simulink model "untitled2"  (R2024b)
settings: Solver=VariableStepAuto  StartTime=0.0  StopTime=10.0  RelTol=1e-3
undefined symbols (not defined in the file): control, Vt, zGround
libraries: uavalgslib x7
settings Model: Creator=USER  LastModifiedBy=USER

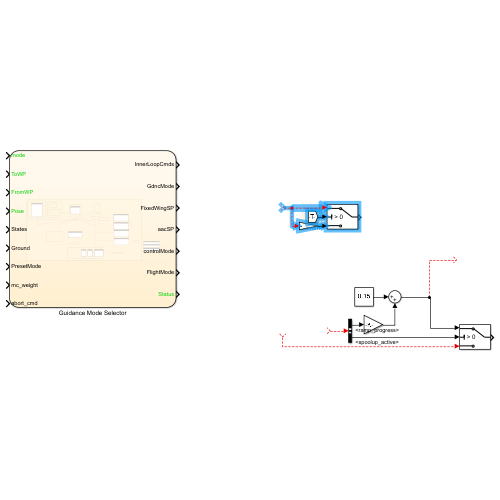
[thumbnail: Simulink's stored preview of the top-level diagram]
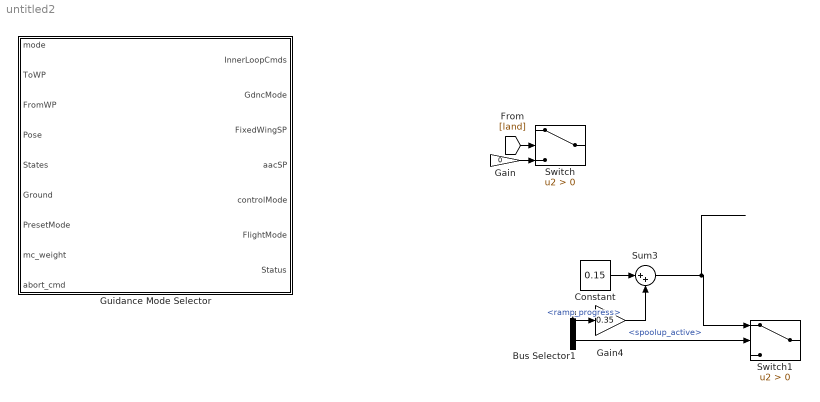
== system untitled2 ==
  Bus Selector1 : BusSelector  OutputSignals=ramp_progress,spoolup_active
  Constant : Constant  Value=0.15
  Gain : Gain  Gain=0
  Gain4 : Gain  Gain=0.35
  Guidance Mode Selector : Stateflow chart  TreatAsAtomicUnit=on
      settings: PortSchema="{\"entries\":[{\"content\":{\"sides\":[{\"content\":{\"connectorIds\":[\"In1\",\"In2\",\"In3\",\"In4\",\"In5\",\"In7\",\"In6\",\"In8\",\"In9\"]},\"type\":\"ConnectorPlacement.EquallySpacedRectSide\",\"uuid\":\"a9cfd0e2-196c-422d-b359-9161a47768c9\"},{\"content\":{\"connectorIds\":[\"Out7\",\"Out2\",\"Out4\",\"Out3\",\"Out5\",\"Out6\",\"Out1\"],\"side\":\"RIGHT\"},\"type\":\"ConnectorPlacement.EquallySpacedRectSide\",\"uuid\":\"4fed41ae-e7cf-4de3-8bdb-9e24e7d8b079\"},{\"content\":{\"side\":\"TOP\"},\"type\":\"ConnectorPlacement.EquallySpacedRectSide\",\"uuid\":\"2d49ff20-2f63-498d-ac9d-820eae01f794\"},{\"content\":{\"side\":\"BOTTOM\"},\"type\":\"ConnectorPlacement.EquallySpacedRectSide\",\"uuid\":\"da24ee44-6e15-4e50-9b36-ff21cb47946d\"}]},\"type\":\"ConnectorPlacement.EquallySpacedConnector\",\"uuid\":\"88d403f4-ad96-40f9-9697-84906f26a8bf\"}],\"packageUris\":[\"http://schema.mathworks.com/mf0/Connector/R2020b\"],\"version\":\"1.0\"}"
  Sum3 : Sum  Inputs=|++
  Switch : Switch  Criteria=u2 > Threshold  SaturateOnIntegerOverflow=off  InputSameDT=off
  Switch1 : Switch  Criteria=u2 > Threshold  SaturateOnIntegerOverflow=off  InputSameDT=off
  wires:
  ? -> Gain/1, Switch/1
  [land] -> Switch/2
  Gain/1 -> Switch/3
  Bus Selector1/2 -> Switch1/2  "<spoolup_active>"
  ? -> Bus Selector1/1
  ? -> Switch1/3
  Sum3/1 -> Switch1/1
  Gain4/1 -> Sum3/2
  Constant/1 -> Sum3/1
  Bus Selector1/1 -> Gain4/1  "<ramp_progress>"

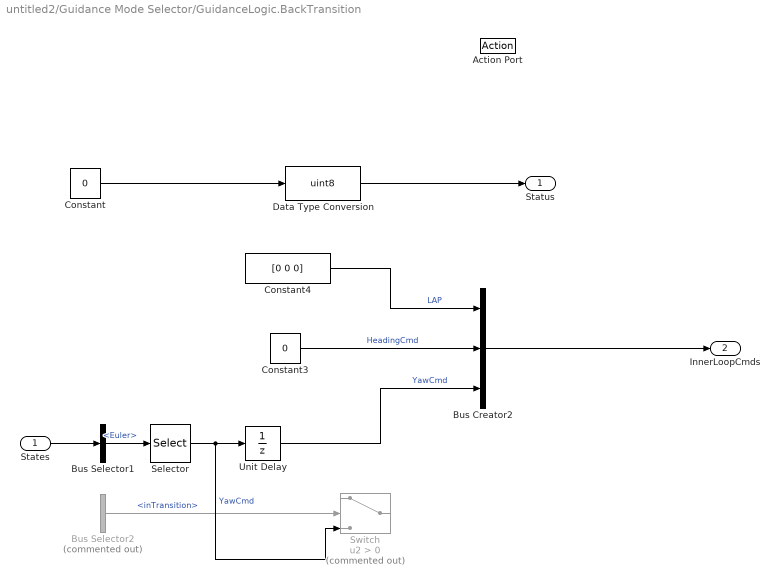
== system untitled2/Guidance Mode Selector/GuidanceLogic.BackTransition ==
  States : Inport  OutDataTypeStr=Bus: StateBus
  Action Port : ActionPort
      settings: CopyFcn=Stateflow.SLINSF.SimulinkMan.removeBlockPreDeleteFcn  PreDeleteFcn=Stateflow.SLINSF.SimulinkMan.unsafePredeleteFcn
  Bus Creator2 : BusCreator  Inputs=3  OutDataTypeStr=Bus: innerLoopCmdsBus  NonVirtualBus=on
  Bus Selector1 : BusSelector  OutputSignals=Euler
  Bus Selector2 : BusSelector  Commented=on  OutputSignals=inTransition
  Constant : Constant  Value=0
  Constant3 : Constant  Value=0
  Constant4 : Constant  Value=[0 0 0]
  Data Type Conversion : DataTypeConversion  OutDataTypeStr=uint8  SaturateOnIntegerOverflow=off  RndMeth=Floor
  Selector : Selector  InputPortWidth=3  IndexOptions=Index vector (dialog)  Indices=3  OutputSizes=1
  Switch : Switch  Commented=on  Criteria=u2 > Threshold  SaturateOnIntegerOverflow=off  InputSameDT=off
  Unit Delay : UnitDelay  SampleTime=-1  HasFrameUpgradeWarning=on
  Status : Outport
  InnerLoopCmds : Outport  Port=2  OutDataTypeStr=Bus: innerLoopCmdsBus
  wires:
  Data Type Conversion/1 -> Status/1
  Constant/1 -> Data Type Conversion/1
  Bus Selector2/1 -> Switch/2  "<inTransition>"
  Constant3/1 -> Bus Creator2/2  "HeadingCmd"
  Unit Delay/1 -> Bus Creator2/3  "YawCmd"
  States/1 -> Bus Selector1/1
  Bus Creator2/1 -> InnerLoopCmds/1
  Constant4/1 -> Bus Creator2/1  "LAP"
  Bus Selector1/1 -> Selector/1  "<Euler>"
  Selector/1 -> Switch/3, Unit Delay/1  "YawCmd"

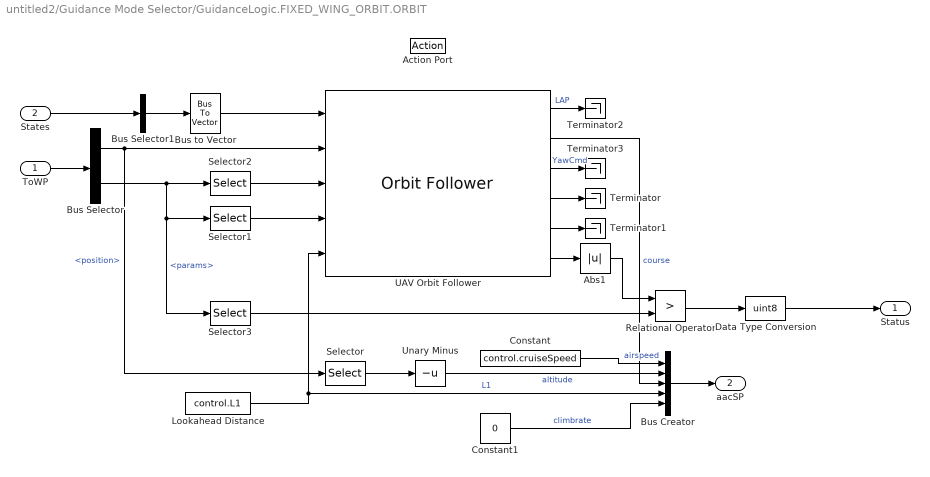
== system untitled2/Guidance Mode Selector/GuidanceLogic.FIXED_WING_ORBIT.ORBIT ==
  ToWP : Inport  OutDataTypeStr=Bus: UAVPathManagerBus
  States : Inport  Port=2
  Action Port : ActionPort
      settings: CopyFcn=Stateflow.SLINSF.SimulinkMan.removeBlockPreDeleteFcn  PreDeleteFcn=Stateflow.SLINSF.SimulinkMan.unsafePredeleteFcn
  Abs1 : Abs  SaturateOnIntegerOverflow=off
  Bus Creator : BusCreator  Inputs=5  OutDataTypeStr=Bus: AAC  NonVirtualBus=on
      settings: InheritFromInputs=off
  Bus Selector : BusSelector  OutputSignals=position,params
  Bus Selector1 : BusSelector  OutputSignals=Xe,course  OutputAsBus=on
  Bus to Vector : BusToVector
  Constant : Constant  Value=control.cruiseSpeed
  Constant1 : Constant  Value=0
  Data Type Conversion : DataTypeConversion  OutDataTypeStr=uint8  SaturateOnIntegerOverflow=off  RndMeth=Floor
  Lookahead Distance : Constant  Value=control.L1  OutDataTypeStr=double
  Relational Operator : RelationalOperator  Operator=>  OutDataTypeStr=boolean  RndMeth=Simplest  InputSameDT=off
  Selector : Selector  InputPortWidth=3  IndexOptions=Index vector (dialog)  Indices=3  OutputSizes=1
  Selector1 : Selector  InputPortWidth=4  IndexOptions=Index vector (dialog)  Indices=2  OutputSizes=1
  Selector2 : Selector  InputPortWidth=4  IndexOptions=Index vector (dialog)  Indices=1  OutputSizes=1
  Selector3 : Selector  InputPortWidth=4  IndexOptions=Index vector (dialog)  Indices=3  OutputSizes=1
  Terminator{,1..3} (4 alike) : Terminator
  UAV Orbit Follower : uavalgslib/Orbit Follower  UAVType=fixed-wing  MinOrbitRadius=control.turningRadius  MinLookaheadDistance=control.L1  ExternalReset=none  ShowCrossTrackErrorOutput=off  ShowNumTurnsOutput=on  SimulateUsing=Code generation
  Unary Minus : UnaryMinus
  Status : Outport
  aacSP : Outport  Port=2
  wires:
  Bus to Vector/1 -> UAV Orbit Follower/1
  Selector2/1 -> UAV Orbit Follower/3
  Bus Selector/1 -> UAV Orbit Follower/2, Selector/1  "<position>"
  ToWP/1 -> Bus Selector/1
  Bus Selector/2 -> Selector1/1, Selector3/1, Selector2/1  "<params>"
  Selector3/1 -> Relational Operator/2
  Relational Operator/1 -> Data Type Conversion/1
  UAV Orbit Follower/4 -> Terminator/1
  UAV Orbit Follower/5 -> Terminator1/1
  Bus Selector1/1 -> Bus to Vector/1
  States/1 -> Bus Selector1/1
  UAV Orbit Follower/1 -> Terminator2/1  "LAP"
  Lookahead Distance/1 -> UAV Orbit Follower/5, Bus Creator/4  "L1"
  Bus Creator/1 -> aacSP/1
  UAV Orbit Follower/2 -> Bus Creator/3  "course"
  Constant/1 -> Bus Creator/1  "airspeed"
  Unary Minus/1 -> Bus Creator/2  "altitude"
  UAV Orbit Follower/3 -> Terminator3/1  "YawCmd"
  Selector/1 -> Unary Minus/1
  UAV Orbit Follower/6 -> Abs1/1
  Abs1/1 -> Relational Operator/1
  Selector1/1 -> UAV Orbit Follower/4
  Constant1/1 -> Bus Creator/5  "climbrate"
  Data Type Conversion/1 -> Status/1

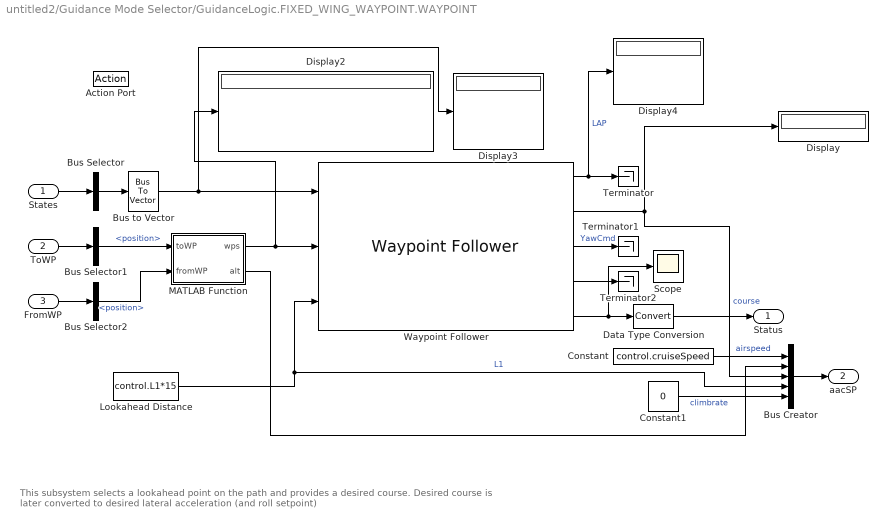
== system untitled2/Guidance Mode Selector/GuidanceLogic.FIXED_WING_WAYPOINT.WAYPOINT ==
  note: This subsystem selects a lookahead point on the path and provides a desired course. Desired course is later converted to desired lateral acceleration (and roll setpoint)
  States : Inport  OutDataTypeStr=Bus: StateBus
  ToWP : Inport  Port=2  OutDataTypeStr=Bus: UAVPathManagerBus
  FromWP : Inport  Port=3  OutDataTypeStr=Bus: UAVPathManagerBus
  Action Port : ActionPort
      settings: CopyFcn=Stateflow.SLINSF.SimulinkMan.removeBlockPreDeleteFcn  PreDeleteFcn=Stateflow.SLINSF.SimulinkMan.unsafePredeleteFcn
  Bus Creator : BusCreator  Inputs=5  OutDataTypeStr=Bus: AAC  NonVirtualBus=on
      settings: InheritFromInputs=off
  Bus Selector : BusSelector  OutputSignals=Xe,course  OutputAsBus=on
  Bus Selector1 : BusSelector  OutputSignals=position
  Bus Selector2 : BusSelector  OutputSignals=position
  Bus to Vector : BusToVector
  Constant : Constant  Value=control.cruiseSpeed
  Constant1 : Constant  Value=0
  Data Type Conversion : DataTypeConversion  SaturateOnIntegerOverflow=off  RndMeth=Floor
  Display{,2..4} (4 alike) : Display
  Lookahead Distance : Constant  Value=control.L1*15  OutDataTypeStr=double
  MATLAB Function : MATLAB Function  TreatAsAtomicUnit=on
  Scope : Scope
  Terminator : Terminator
  Terminator1 : Terminator
  Terminator2 : Terminator
  Waypoint Follower : uavalgslib/Waypoint Follower  UAVType=fixed-wing  StartFrom=first  TransitionRadiusSource=internal  TransitionRadius=FWControl.transitionRadius  MinLookaheadDistance=control.L1  HoverAtLastWaypoint=off  YawInput=off  ShowCrossTrackErrorOutput=off  ShowStatusOutput=on  SimulateUsing=Code generation
  Status : Outport
  aacSP : Outport  Port=2
  wires:
  Lookahead Distance/1 -> Waypoint Follower/3, Bus Creator/4  "L1"
  Waypoint Follower/1 -> Display4/1, Terminator/1  "LAP"
  Waypoint Follower/3 -> Terminator1/1  "YawCmd"
  Waypoint Follower/4 -> Terminator2/1
  Constant/1 -> Bus Creator/1  "airspeed"
  States/1 -> Bus Selector/1
  Bus Selector/1 -> Bus to Vector/1
  Waypoint Follower/5 -> Scope/1, Data Type Conversion/1
  Data Type Conversion/1 -> Status/1
  Bus Creator/1 -> aacSP/1
  ToWP/1 -> Bus Selector1/1
  FromWP/1 -> Bus Selector2/1
  Bus Selector1/1 -> MATLAB Function/1(toWP)  "<position>"
  Bus Selector2/1 -> MATLAB Function/2(fromWP)  "<position>"
  MATLAB Function/2(alt) -> Bus Creator/2
  Waypoint Follower/2 -> Display/1, Bus Creator/3  "course"
  Constant1/1 -> Bus Creator/5  "climbrate"
  Bus to Vector/1 -> Display3/1, Waypoint Follower/1
  MATLAB Function/1(wps) -> Display2/1, Waypoint Follower/2

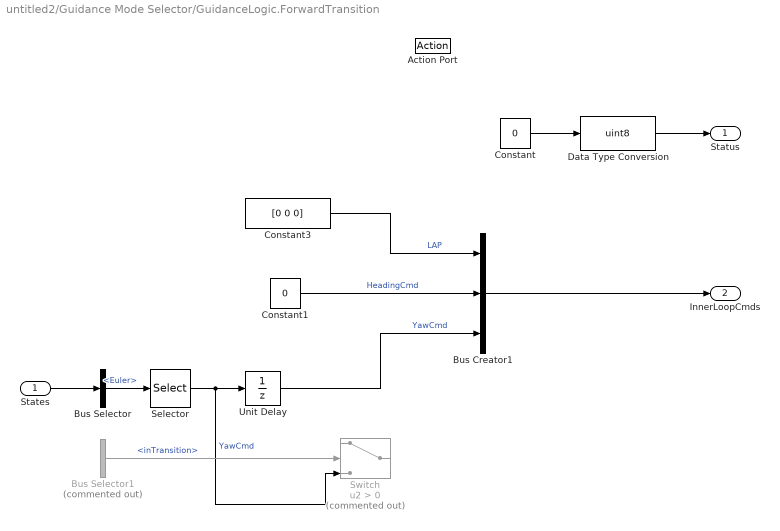
== system untitled2/Guidance Mode Selector/GuidanceLogic.ForwardTransition ==
  States : Inport  OutDataTypeStr=Bus: StateBus
  Action Port : ActionPort
      settings: CopyFcn=Stateflow.SLINSF.SimulinkMan.removeBlockPreDeleteFcn  PreDeleteFcn=Stateflow.SLINSF.SimulinkMan.unsafePredeleteFcn
  Bus Creator1 : BusCreator  Inputs=3  OutDataTypeStr=Bus: innerLoopCmdsBus  NonVirtualBus=on
  Bus Selector : BusSelector  OutputSignals=Euler
  Bus Selector1 : BusSelector  Commented=on  OutputSignals=inTransition
  Constant : Constant  Value=0
  Constant1 : Constant  Value=0
  Constant3 : Constant  Value=[0 0 0]
  Data Type Conversion : DataTypeConversion  OutDataTypeStr=uint8  SaturateOnIntegerOverflow=off  RndMeth=Floor
  Selector : Selector  InputPortWidth=3  IndexOptions=Index vector (dialog)  Indices=3  OutputSizes=1
  Switch : Switch  Commented=on  Criteria=u2 > Threshold  SaturateOnIntegerOverflow=off  InputSameDT=off
  Unit Delay : UnitDelay  SampleTime=-1  HasFrameUpgradeWarning=on
  Status : Outport
  InnerLoopCmds : Outport  Port=2  OutDataTypeStr=Bus: innerLoopCmdsBus
  wires:
  Bus Creator1/1 -> InnerLoopCmds/1
  Constant1/1 -> Bus Creator1/2  "HeadingCmd"
  Selector/1 -> Switch/3, Unit Delay/1  "YawCmd"
  Data Type Conversion/1 -> Status/1
  Constant/1 -> Data Type Conversion/1
  Constant3/1 -> Bus Creator1/1  "LAP"
  States/1 -> Bus Selector/1
  Bus Selector/1 -> Selector/1  "<Euler>"
  Bus Selector1/1 -> Switch/2  "<inTransition>"
  Unit Delay/1 -> Bus Creator1/3  "YawCmd"

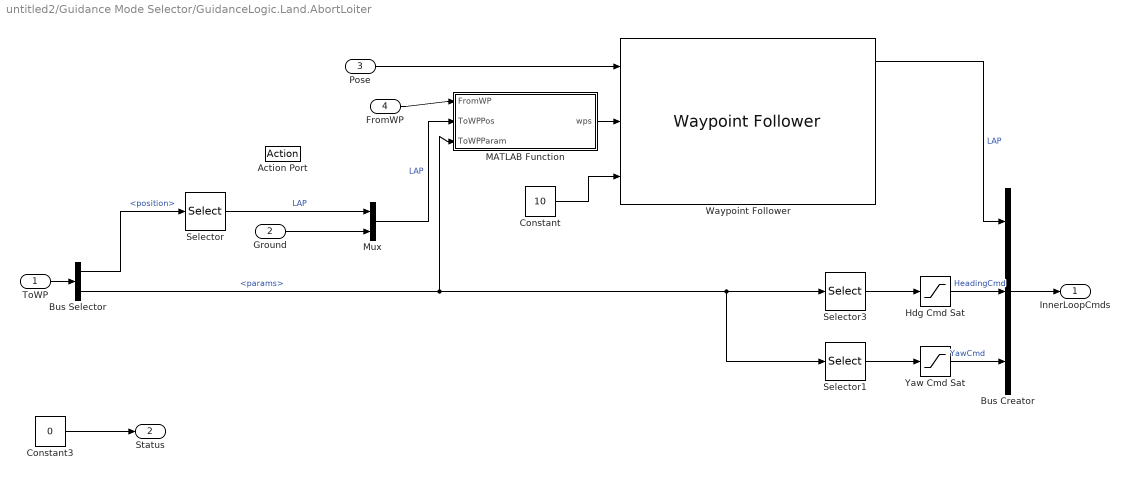
== system untitled2/Guidance Mode Selector/GuidanceLogic.Land.AbortLoiter ==
  ToWP : Inport  OutDataTypeStr=Bus: UAVPathManagerBus
  Ground : Inport  Port=2
  Pose : Inport  Port=3
  FromWP : Inport  Port=4  OutDataTypeStr=Bus: UAVPathManagerBus
  Action Port : ActionPort
      settings: CopyFcn=Stateflow.SLINSF.SimulinkMan.removeBlockPreDeleteFcn  PreDeleteFcn=Stateflow.SLINSF.SimulinkMan.unsafePredeleteFcn
  Bus Creator : BusCreator  Inputs=3  OutDataTypeStr=Bus: innerLoopCmdsBus  NonVirtualBus=on
      settings: InheritFromInputs=off
  Bus Selector : BusSelector  OutputSignals=position,params
  Constant : Constant  Value=10
  Constant3 : Constant  Value=0  OutDataTypeStr=uint8
  Hdg Cmd Sat : Saturate  UpperLimit=pi  LowerLimit=-pi
      settings: AttributesFormatString=[%<UpperLimit> %<LowerLimit>]
  MATLAB Function : MATLAB Function  TreatAsAtomicUnit=on
  Mux : Mux  Inputs=2
  Selector : Selector  InputPortWidth=3  IndexOptions=Index vector (dialog)  Indices=[1 2]  OutputSizes=1
  Selector1 : Selector  InputPortWidth=4  IndexOptions=Index vector (dialog)  Indices=4  OutputSizes=1
  Selector3 : Selector  InputPortWidth=4  IndexOptions=Index vector (dialog)  Indices=4  OutputSizes=1
  Waypoint Follower : uavalgslib/Waypoint Follower  UAVType=multirotor  StartFrom=first  TransitionRadiusSource=internal  TransitionRadius=1  MinLookaheadDistance=0.1  HoverAtLastWaypoint=on  YawInput=on  ShowCrossTrackErrorOutput=off  ShowStatusOutput=off  SimulateUsing=Code generation
  Yaw Cmd Sat : Saturate  UpperLimit=pi  LowerLimit=-pi
      settings: AttributesFormatString=[%<UpperLimit> %<LowerLimit>]
  InnerLoopCmds : Outport  OutDataTypeStr=Bus: innerLoopCmdsBus
  Status : Outport  Port=2
  wires:
  Bus Creator/1 -> InnerLoopCmds/1
  Bus Selector/1 -> Selector/1  "<position>"
  Yaw Cmd Sat/1 -> Bus Creator/3  "YawCmd"
  Hdg Cmd Sat/1 -> Bus Creator/2  "HeadingCmd"
  ToWP/1 -> Bus Selector/1
  Selector1/1 -> Yaw Cmd Sat/1
  Selector3/1 -> Hdg Cmd Sat/1
  Selector/1 -> Mux/1  "LAP"
  Bus Selector/2 -> MATLAB Function/3(ToWPParam), Selector1/1, Selector3/1  "<params>"
  Ground/1 -> Mux/2
  Constant3/1 -> Status/1
  Mux/1 -> MATLAB Function/2(ToWPPos)  "LAP"
  FromWP/1 -> MATLAB Function/1(FromWP)
  Pose/1 -> Waypoint Follower/1
  MATLAB Function/1(wps) -> Waypoint Follower/2
  Constant/1 -> Waypoint Follower/3
  Waypoint Follower/1 -> Bus Creator/1  "LAP"

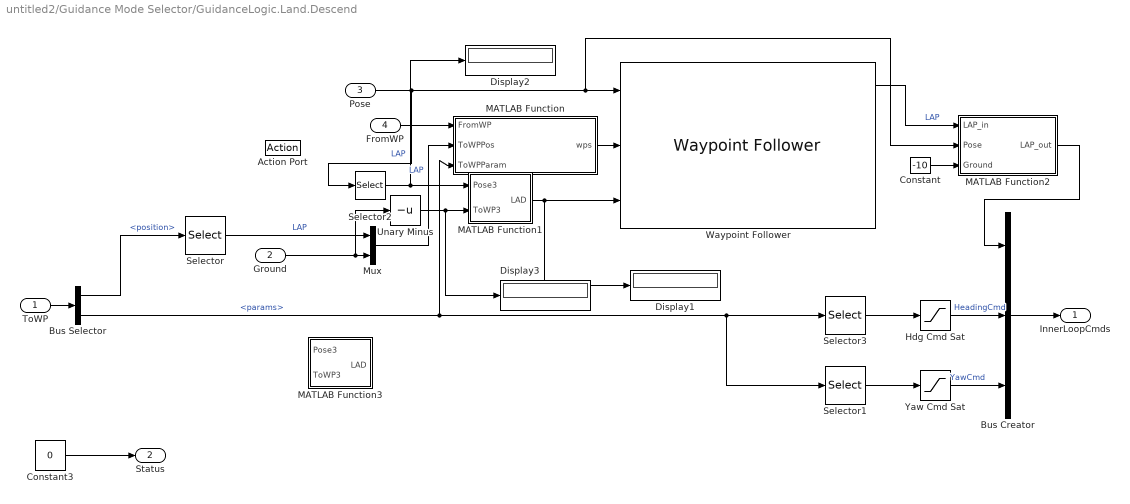
== system untitled2/Guidance Mode Selector/GuidanceLogic.Land.Descend ==
  ToWP : Inport  OutDataTypeStr=Bus: UAVPathManagerBus
  Ground : Inport  Port=2
  Pose : Inport  Port=3
  FromWP : Inport  Port=4  OutDataTypeStr=Bus: UAVPathManagerBus
  Action Port : ActionPort
      settings: CopyFcn=Stateflow.SLINSF.SimulinkMan.removeBlockPreDeleteFcn  PreDeleteFcn=Stateflow.SLINSF.SimulinkMan.unsafePredeleteFcn
  Bus Creator : BusCreator  Inputs=3  OutDataTypeStr=Bus: innerLoopCmdsBus  NonVirtualBus=on
      settings: InheritFromInputs=off
  Bus Selector : BusSelector  OutputSignals=position,params
  Constant : Constant  Value=-10
  Constant3 : Constant  Value=0  OutDataTypeStr=uint8
  Display1 : Display
  Display2 : Display
  Display3 : Display
  Hdg Cmd Sat : Saturate  UpperLimit=pi  LowerLimit=-pi
      settings: AttributesFormatString=[%<UpperLimit> %<LowerLimit>]
  MATLAB Function : MATLAB Function  TreatAsAtomicUnit=on
  MATLAB Function1 : MATLAB Function  TreatAsAtomicUnit=on
  MATLAB Function2 : MATLAB Function  TreatAsAtomicUnit=on
  MATLAB Function3 : MATLAB Function  TreatAsAtomicUnit=on
  Mux : Mux  Inputs=2
  Selector : Selector  InputPortWidth=3  IndexOptions=Index vector (dialog)  Indices=[1 2]  OutputSizes=1
  Selector1 : Selector  InputPortWidth=4  IndexOptions=Index vector (dialog)  Indices=4  OutputSizes=1
  Selector2 : Selector  InputPortWidth=4  IndexOptions=Index vector (dialog)  Indices=3  OutputSizes=1
  Selector3 : Selector  InputPortWidth=4  IndexOptions=Index vector (dialog)  Indices=4  OutputSizes=1
  Unary Minus : UnaryMinus
  Waypoint Follower : uavalgslib/Waypoint Follower  UAVType=multirotor  StartFrom=first  TransitionRadiusSource=internal  TransitionRadius=1  MinLookaheadDistance=0.1  HoverAtLastWaypoint=on  YawInput=on  ShowCrossTrackErrorOutput=off  ShowStatusOutput=off  SimulateUsing=Code generation
  Yaw Cmd Sat : Saturate  UpperLimit=pi  LowerLimit=-pi
      settings: AttributesFormatString=[%<UpperLimit> %<LowerLimit>]
  InnerLoopCmds : Outport  OutDataTypeStr=Bus: innerLoopCmdsBus
  Status : Outport  Port=2
  wires:
  Bus Creator/1 -> InnerLoopCmds/1
  Bus Selector/1 -> Selector/1  "<position>"
  Yaw Cmd Sat/1 -> Bus Creator/3  "YawCmd"
  Hdg Cmd Sat/1 -> Bus Creator/2  "HeadingCmd"
  ToWP/1 -> Bus Selector/1
  Selector1/1 -> Yaw Cmd Sat/1
  Selector3/1 -> Hdg Cmd Sat/1
  Selector/1 -> Mux/1  "LAP"
  Bus Selector/2 -> MATLAB Function/3(ToWPParam), Selector1/1, Selector3/1  "<params>"
  Ground/1 -> Unary Minus/1, Mux/2
  Constant3/1 -> Status/1
  Mux/1 -> MATLAB Function/2(ToWPPos)  "LAP"
  FromWP/1 -> MATLAB Function/1(FromWP)
  Pose/1 -> Selector2/1, MATLAB Function2/2(Pose), Waypoint Follower/1
  MATLAB Function/1(wps) -> Waypoint Follower/2
  Selector2/1 -> MATLAB Function1/1(Pose3), Display2/1  "LAP"
  MATLAB Function1/1(LAD) -> Waypoint Follower/3, Display1/1
  Waypoint Follower/1 -> MATLAB Function2/1(LAP_in)  "LAP"
  MATLAB Function2/1(LAP_out) -> Bus Creator/1
  Constant/1 -> MATLAB Function2/3(Ground)
  Unary Minus/1 -> Display3/1, MATLAB Function1/2(ToWP3)

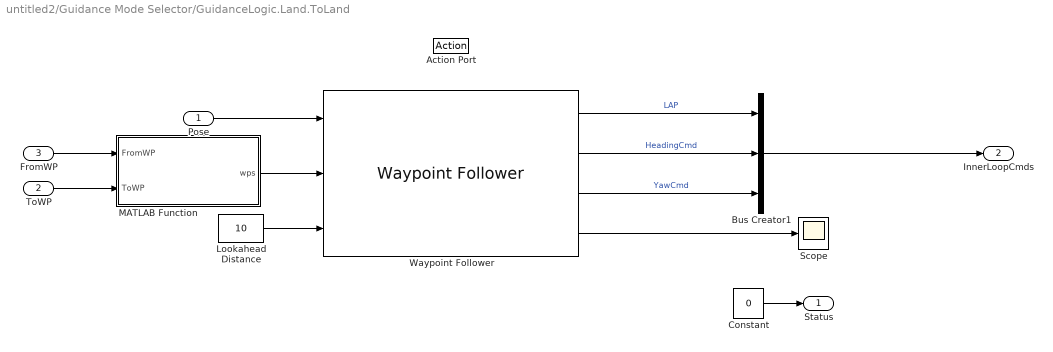
== system untitled2/Guidance Mode Selector/GuidanceLogic.Land.ToLand ==
  Pose : Inport
  ToWP : Inport  Port=2  OutDataTypeStr=Bus: UAVPathManagerBus
  FromWP : Inport  Port=3  OutDataTypeStr=Bus: UAVPathManagerBus
  Action Port : ActionPort
      settings: CopyFcn=Stateflow.SLINSF.SimulinkMan.removeBlockPreDeleteFcn  PreDeleteFcn=Stateflow.SLINSF.SimulinkMan.unsafePredeleteFcn
  Bus Creator1 : BusCreator  Inputs=3  OutDataTypeStr=Bus: innerLoopCmdsBus  NonVirtualBus=on
  Constant : Constant  Value=0  OutDataTypeStr=uint8
  Lookahead Distance : Constant  Value=10  OutDataTypeStr=double
  MATLAB Function : MATLAB Function  TreatAsAtomicUnit=on
  Scope : Scope
  Waypoint Follower : uavalgslib/Waypoint Follower  UAVType=multirotor  StartFrom=first  TransitionRadiusSource=internal  TransitionRadius=1  MinLookaheadDistance=0.1  HoverAtLastWaypoint=on  YawInput=on  ShowCrossTrackErrorOutput=off  ShowStatusOutput=off  SimulateUsing=Code generation
  Status : Outport
  InnerLoopCmds : Outport  Port=2  OutDataTypeStr=Bus: innerLoopCmdsBus
  wires:
  Constant/1 -> Status/1
  MATLAB Function/1(wps) -> Waypoint Follower/2
  Lookahead Distance/1 -> Waypoint Follower/3
  Bus Creator1/1 -> InnerLoopCmds/1
  ToWP/1 -> MATLAB Function/2(ToWP)
  Waypoint Follower/2 -> Bus Creator1/2  "HeadingCmd"
  FromWP/1 -> MATLAB Function/1(FromWP)
  Waypoint Follower/4 -> Scope/1
  Pose/1 -> Waypoint Follower/1
  Waypoint Follower/3 -> Bus Creator1/3  "YawCmd"
  Waypoint Follower/1 -> Bus Creator1/1  "LAP"

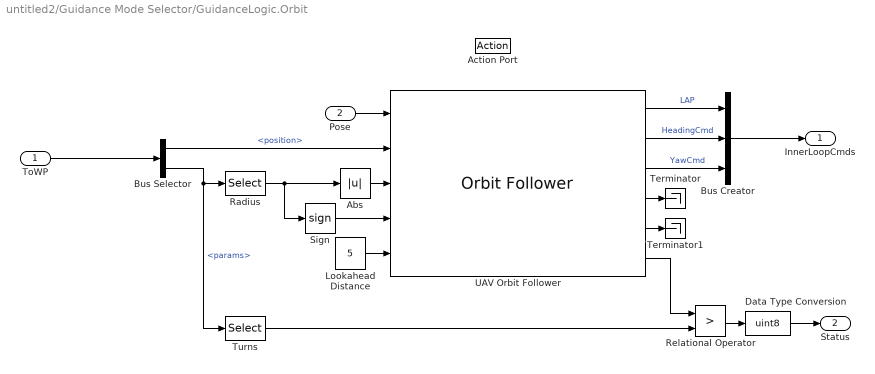
== system untitled2/Guidance Mode Selector/GuidanceLogic.Orbit ==
  ToWP : Inport  OutDataTypeStr=Bus: UAVPathManagerBus
  Pose : Inport  Port=2
  Action Port : ActionPort
      settings: CopyFcn=Stateflow.SLINSF.SimulinkMan.removeBlockPreDeleteFcn  PreDeleteFcn=Stateflow.SLINSF.SimulinkMan.unsafePredeleteFcn
  Abs : Abs  SaturateOnIntegerOverflow=off
  Bus Creator : BusCreator  Inputs=3  OutDataTypeStr=Bus: innerLoopCmdsBus  NonVirtualBus=on
  Bus Selector : BusSelector  OutputSignals=position,params
  Data Type Conversion : DataTypeConversion  OutDataTypeStr=uint8  SaturateOnIntegerOverflow=off  RndMeth=Floor
  Lookahead Distance : Constant  Value=5  OutDataTypeStr=double
  Radius : Selector  InputPortWidth=4  IndexOptions=Index vector (dialog)  Indices=[3]  OutputSizes=1
  Relational Operator : RelationalOperator  Operator=>  OutDataTypeStr=boolean  RndMeth=Simplest  InputSameDT=off
  Sign : Signum  ZeroCross=off
  Terminator : Terminator
  Terminator1 : Terminator
  Turns : Selector  InputPortWidth=4  IndexOptions=Index vector (dialog)  Indices=[1]  OutputSizes=1
  UAV Orbit Follower : uavalgslib/Orbit Follower  UAVType=multirotor  MinOrbitRadius=1  MinLookaheadDistance=0.1  ExternalReset=none  ShowCrossTrackErrorOutput=off  ShowNumTurnsOutput=on  SimulateUsing=Code generation
  InnerLoopCmds : Outport  OutDataTypeStr=Bus: innerLoopCmdsBus
  Status : Outport  Port=2
  wires:
  Pose/1 -> UAV Orbit Follower/1
  Lookahead Distance/1 -> UAV Orbit Follower/5
  Abs/1 -> UAV Orbit Follower/3
  Bus Selector/1 -> UAV Orbit Follower/2  "<position>"
  ToWP/1 -> Bus Selector/1
  Bus Creator/1 -> InnerLoopCmds/1
  UAV Orbit Follower/2 -> Bus Creator/2  "HeadingCmd"
  UAV Orbit Follower/3 -> Bus Creator/3  "YawCmd"
  Bus Selector/2 -> Turns/1, Radius/1  "<params>"
  Radius/1 -> Abs/1, Sign/1
  Sign/1 -> UAV Orbit Follower/4
  Relational Operator/1 -> Data Type Conversion/1
  Turns/1 -> Relational Operator/2
  Data Type Conversion/1 -> Status/1
  UAV Orbit Follower/6 -> Relational Operator/1
  UAV Orbit Follower/4 -> Terminator/1
  UAV Orbit Follower/5 -> Terminator1/1
  UAV Orbit Follower/1 -> Bus Creator/1  "LAP"

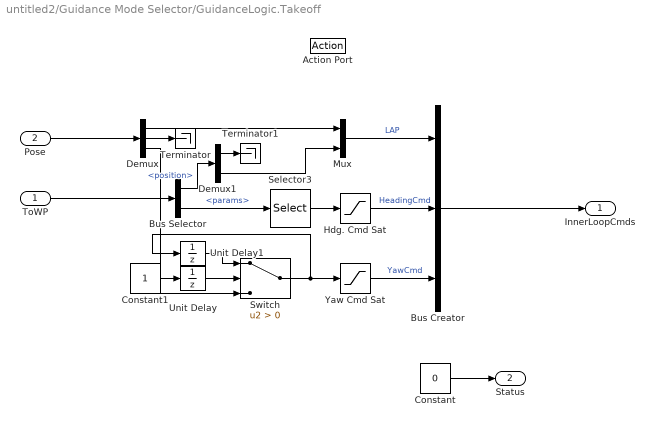
== system untitled2/Guidance Mode Selector/GuidanceLogic.Takeoff ==
  ToWP : Inport  OutDataTypeStr=Bus: UAVPathManagerBus
  Pose : Inport  Port=2
  Action Port : ActionPort
      settings: CopyFcn=Stateflow.SLINSF.SimulinkMan.removeBlockPreDeleteFcn  PreDeleteFcn=Stateflow.SLINSF.SimulinkMan.unsafePredeleteFcn
  Bus Creator : BusCreator  Inputs=3  OutDataTypeStr=Bus: innerLoopCmdsBus  NonVirtualBus=on
      settings: InheritFromInputs=off
  Bus Selector : BusSelector  OutputSignals=position,params
  Constant : Constant  Value=0  OutDataTypeStr=uint8
  Constant1 : Constant
  Demux : Demux  Outputs=[2 1 1]
  Demux1 : Demux  Outputs=[2 1]
  Hdg. Cmd Sat : Saturate  UpperLimit=pi  LowerLimit=-pi
      settings: AttributesFormatString=[%<UpperLimit> %<LowerLimit>]
  Mux : Mux  Inputs=2
  Selector3 : Selector  InputPortWidth=4  IndexOptions=Index vector (dialog)  Indices=1  OutputSizes=1
  Switch : Switch  Criteria=u2 > Threshold  SaturateOnIntegerOverflow=off  InputSameDT=off
  Terminator : Terminator
  Terminator1 : Terminator
  Unit Delay : UnitDelay  SampleTime=-1  HasFrameUpgradeWarning=on
  Unit Delay1 : UnitDelay  SampleTime=-1  HasFrameUpgradeWarning=on
  Yaw Cmd Sat : Saturate  UpperLimit=pi  LowerLimit=-pi
      settings: AttributesFormatString=[%<UpperLimit> %<LowerLimit>]
  InnerLoopCmds : Outport  OutDataTypeStr=Bus: innerLoopCmdsBus
  Status : Outport  Port=2
  wires:
  Hdg. Cmd Sat/1 -> Bus Creator/2  "HeadingCmd"
  Bus Creator/1 -> InnerLoopCmds/1
  Constant/1 -> Status/1
  Pose/1 -> Demux/1
  Yaw Cmd Sat/1 -> Bus Creator/3  "YawCmd"
  ToWP/1 -> Bus Selector/1
  Bus Selector/2 -> Selector3/1  "<params>"
  Demux/1 -> Mux/1
  Bus Selector/1 -> Demux1/1  "<position>"
  Demux/2 -> Terminator/1
  Demux1/1 -> Terminator1/1
  Selector3/1 -> Hdg. Cmd Sat/1
  Demux1/2 -> Mux/2
  Mux/1 -> Bus Creator/1  "LAP"
  Constant1/1 -> Unit Delay/1
  Switch/1 -> Unit Delay1/1, Yaw Cmd Sat/1
  Demux/3 -> Switch/3
  Unit Delay/1 -> Switch/2
  Unit Delay1/1 -> Switch/1

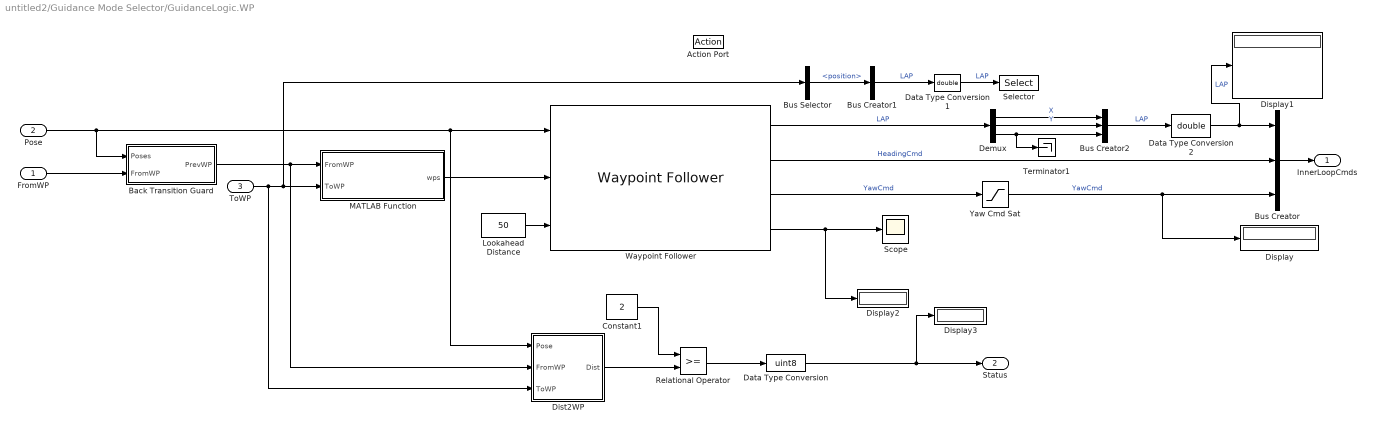
== system untitled2/Guidance Mode Selector/GuidanceLogic.WP ==
  FromWP : Inport  OutDataTypeStr=Bus: UAVPathManagerBus
  Pose : Inport  Port=2
  ToWP : Inport  Port=3  OutDataTypeStr=Bus: UAVPathManagerBus
  Action Port : ActionPort
      settings: CopyFcn=Stateflow.SLINSF.SimulinkMan.removeBlockPreDeleteFcn  PreDeleteFcn=Stateflow.SLINSF.SimulinkMan.unsafePredeleteFcn
  Back Transition Guard : Subsystem
  Bus Creator : BusCreator  Inputs=3  OutDataTypeStr=Bus: innerLoopCmdsBus  NonVirtualBus=on
  Bus Creator1 : BusCreator  Inputs=1
  Bus Creator2 : BusCreator  Inputs=3
  Bus Selector : BusSelector  OutputSignals=position
  Constant1 : Constant  Value=2
  Data Type Conversion : DataTypeConversion  OutDataTypeStr=uint8  SaturateOnIntegerOverflow=off  RndMeth=Floor
  Data Type Conversion1 : DataTypeConversion  OutDataTypeStr=double  SaturateOnIntegerOverflow=off  RndMeth=Floor
  Data Type Conversion2 : DataTypeConversion  OutDataTypeStr=double  SaturateOnIntegerOverflow=off  RndMeth=Floor
  Demux : Demux  Outputs=3
  Display{,1..3} (4 alike) : Display
  Dist2WP : Subsystem
  Lookahead Distance : Constant  Value=50  OutDataTypeStr=double
  MATLAB Function : MATLAB Function  TreatAsAtomicUnit=on
  Relational Operator : RelationalOperator  OutDataTypeStr=boolean  RndMeth=Simplest  InputSameDT=off
  Scope : Scope
  Selector : Selector  InputPortWidth=3  IndexOptions=Index vector (dialog)  Indices=3  OutputSizes=1
  Terminator1 : Terminator
  Waypoint Follower : uavalgslib/Waypoint Follower  UAVType=multirotor  StartFrom=closest  TransitionRadiusSource=internal  TransitionRadius=R_WAYPOINTTRANSITION  MinLookaheadDistance=0.1  HoverAtLastWaypoint=off  YawInput=on  ShowCrossTrackErrorOutput=off  ShowStatusOutput=off  SimulateUsing=Code generation
  Yaw Cmd Sat : Saturate  UpperLimit=pi  LowerLimit=-pi
      settings: AttributesFormatString=[%<UpperLimit> %<LowerLimit>]
  InnerLoopCmds : Outport  OutDataTypeStr=Bus: innerLoopCmdsBus
  Status : Outport  Port=2
  wires:
  Data Type Conversion/1 -> Display3/1, Status/1
  Bus Creator/1 -> InnerLoopCmds/1
  ToWP/1 -> Dist2WP/3(ToWP), Bus Selector/1, MATLAB Function/2(ToWP)
  MATLAB Function/1(wps) -> Waypoint Follower/2
  Waypoint Follower/2 -> Bus Creator/2  "HeadingCmd"
  Waypoint Follower/4 -> Display2/1, Scope/1
  Dist2WP/1(Dist) -> Relational Operator/2
  FromWP/1 -> Back Transition Guard/2(FromWP)
  Relational Operator/1 -> Data Type Conversion/1
  Back Transition Guard/1(PrevWP) -> Dist2WP/2(FromWP), MATLAB Function/1(FromWP)
  Pose/1 -> Back Transition Guard/1(Poses), Waypoint Follower/1, Dist2WP/1(Pose)
  Lookahead Distance/1 -> Waypoint Follower/3
  Waypoint Follower/3 -> Yaw Cmd Sat/1  "YawCmd"
  Constant1/1 -> Relational Operator/1
  Bus Creator1/1 -> Data Type Conversion1/1  "LAP"
  Waypoint Follower/1 -> Demux/1  "LAP"
  Demux/3 -> Terminator1/1, Bus Creator2/3
  Data Type Conversion1/1 -> Selector/1  "LAP"
  Demux/1 -> Bus Creator2/1  "X"
  Demux/2 -> Bus Creator2/2  "Y"
  Bus Creator2/1 -> Data Type Conversion2/1  "LAP"
  Data Type Conversion2/1 -> Display1/1, Bus Creator/1  "LAP"
  Bus Selector/1 -> Bus Creator1/1  "<position>"
  Yaw Cmd Sat/1 -> Display/1, Bus Creator/3  "YawCmd"

== system untitled2/Guidance Mode Selector/GuidanceLogic.WP/Back Transition Guard ==
  note: Set previous waypoint to current location if the UAV has just exited back transition
  Poses : Inport
  FromWP : Inport  Port=2
  Bus Selector : BusSelector  OutputSignals=mode
  Bus Selector1 : BusSelector  OutputSignals=position,params,mode
  Constant : Constant  Value=6
  Equal : RelationalOperator  Operator===  OutDataTypeStr=boolean  RndMeth=Simplest  InputSameDT=off
  Switch : Switch  Criteria=u2 > Threshold  SaturateOnIntegerOverflow=off  InputSameDT=off
  Triggered Subsystem : Subsystem  TreatAsAtomicUnit=on
  Out Bus Element2 : Outport  PortName=PrevWP  Element=mode
  Out Bus Element : Outport  PortName=PrevWP  Element=position
  Out Bus Element1 : Outport  PortName=PrevWP  Element=params
  wires:
  FromWP/1 -> Bus Selector1/1, Bus Selector/1
  Bus Selector/1 -> Equal/2  "<mode>"
  Constant/1 -> Equal/1
  Equal/1 -> Switch/2, Triggered Subsystem/Trigger
  Poses/1 -> Triggered Subsystem/1(Poses)
  Triggered Subsystem/1(HoldPositionValue) -> Switch/1
  Switch/1 -> Out Bus Element/1
  Bus Selector1/2 -> Out Bus Element1/1  "<params>"
  Bus Selector1/3 -> Out Bus Element2/1  "<mode>"
  Bus Selector1/1 -> Switch/3  "<position>"

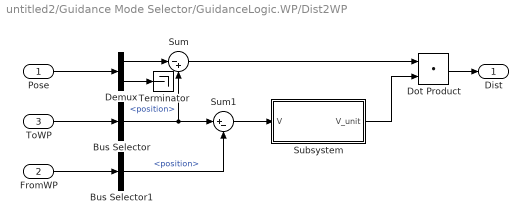
== system untitled2/Guidance Mode Selector/GuidanceLogic.WP/Dist2WP ==
  Pose : Inport
  FromWP : Inport  Port=2
  ToWP : Inport  Port=3
  Bus Selector : BusSelector  OutputSignals=position
  Bus Selector1 : BusSelector  OutputSignals=position
  Demux : Demux  Outputs=[3 1]
  Dot Product : DotProduct  OutDataTypeStr=Inherit: Inherit via internal rule
  Subsystem : Subsystem
  Sum : Sum  Inputs=|-+
  Sum1 : Sum  Inputs=|+-
  Terminator : Terminator
  Dist : Outport
  wires:
  Sum1/1 -> Subsystem/1(V)
  Demux/2 -> Terminator/1
  Bus Selector/1 -> Sum/2, Sum1/1  "<position>"
  Demux/1 -> Sum/1
  Bus Selector1/1 -> Sum1/2  "<position>"
  Sum/1 -> Dot Product/1
  Subsystem/1(V_unit) -> Dot Product/2
  Pose/1 -> Demux/1
  Dot Product/1 -> Dist/1
  ToWP/1 -> Bus Selector/1
  FromWP/1 -> Bus Selector1/1

== system untitled2/Guidance Mode Selector/GuidanceLogic.WP/Back Transition Guard/Triggered Subsystem ==
  Poses : Inport
  Trigger : TriggerPort  VariantControl=(inherit)
  Reshape : Reshape  OutputDimensionality=Customize  OutputDimensions=[3,1]
  Selector : Selector  InputPortWidth=4  IndexOptions=Index vector (dialog)  Indices=[1 2 3]  OutputSizes=1
  HoldPositionValue : Outport
  wires:
  Poses/1 -> Selector/1
  Selector/1 -> Reshape/1
  Reshape/1 -> HoldPositionValue/1

== system untitled2/Guidance Mode Selector/GuidanceLogic.WP/Dist2WP/Subsystem ==
  V : Inport
  Dot Product1 : DotProduct  OutDataTypeStr=Inherit: Inherit via internal rule
  Product : Product  Inputs=*/
  Saturation : Saturate  UpperLimit=inf  LowerLimit=0.00001
  Sqrt : Sqrt
  V_unit : Outport
  wires:
  V/1 -> Dot Product1/2, Dot Product1/1, Product/1
  Sqrt/1 -> Product/2
  Dot Product1/1 -> Saturation/1
  Saturation/1 -> Sqrt/1
  Product/1 -> V_unit/1

== stateflow chart untitled2/Guidance Mode Selector ==
  settings: updateMethod=DISCRETE
  state GuidanceLogic
    state FIXED_WING_WAYPOINT
      en:
      controlMode.airspeedAltitude = 1;
      controlMode.attitude = 1;
      controlMode.lateralGuidance = 1;
      state WAYPOINT
    state FIXED_WING_ENTRY
      state Stabilize
        en:
        FlightMode=flightState.FixedWing;
        controlMode.attitude = 1;
        controlMode.airspeedAltitude = 0;
        controlMode.lateralGuidance = 0;
        %Transition once done.
        FixedWingSP.yaw = 0;
        FixedWingSP.pitch = 0;
        FixedWingSP.roll = 0;
        FixedWingSP.airspeed=14;
        Status= uint8(0);
      state FIXEDWINGFLIGHT
        en:
        % Control mode
        controlMode.airspeedAltitude = 1;
        controlMode.attitude = 1;
        controlMode.lateralGuidance = 1;
        % Setpoint init
        aacSP.L1 = 25;
        aacSP.airspeed = 14;
        aacSP.altitude = 0;
        aacSP.course=0;
      (default) -> Stabilize
      Stabilize -> FIXEDWINGFLIGHT : after(0.5,sec)
    state Start
      en:
      %Set Flight mode to hover
      FlightMode=PresetMode;
      %Set default settings
      % Control mode
      controlMode.airspeedAltitude = 1;
      controlMode.attitude = 1;
      controlMode.lateralGuidance = 0;
      controlMode.TransitionCondition = 0;
      controlMode.BackTransitionCondition=0;
      controlMode.land = 1;
      % Setpoint init
      FixedWingSP.yaw = 0;
      FixedWingSP.pitch = 0;
      FixedWingSP.roll = 0;
      FixedWingSP.airspeed=14;
      aacSP.L1 = 25;
      aacSP.airspeed = 14;
      aacSP.altitude = 0;
      aacSP.course=0;
      InnerLoopCmds.YawCmd=0;
    state FIXED_WING_ORBIT
      en:
      controlMode.airspeedAltitude = 1;
      controlMode.attitude = 1;
      controlMode.lateralGuidance = 1;
      state ORBIT
    state HOVER_ENTRY
      en:
      FlightMode=flightState.Hover;
      controlMode.inTransition=0;
    state Takeoff
    state RAMPUP
      en:
      ramp_progress=0;
      during: ramp_progress =  min(ramp_progress + 0.005/3.0, 1.0);
      controlMode.ramp_progress = ramp_progress;
      ex:
      controlMode.spoolup_active = 0;
    state SPOOLUP
      en:
      spoolup_timer =0;
      controlMode.spoolup_active = 1;
      controlMode.ramp_progress = 0;
      during:
      spoolup_timer = spoolup_timer + 0.005;
    state WP
    state Orbit
    state PreTransition
      en:
      FlightMode=flightState.FixedWing;
      controlMode.airspeedAltitude = 1;
      controlMode.attitude = 1;
      controlMode.lateralGuidance = 1;
      % Setpoint init
      aacSP.L1 = 25;
      aacSP.airspeed = 14;
      aacSP.altitude = altitudeHold;
      aacSP.course=courseHold;
    state BackTransition
    state ForwardTransition
    state FWCOMPLETE
      Status=uint8(1);
      controlMode.TransitionCondition=uint8(1);
    state BackCOMPLETE
      Status=uint8(1);
      controlMode.BackTransitionCondition=uint8(1)
    state Land
      state ToLand
      state AbortLoiter
      state Descend
      (default) -> ToLand
      Descend -> AbortLoiter : [abort_cmd == 1]
      ToLand -> Descend : [(norm(Pose(1:2)-ToWP.position(1:2)) <= 10)]
      AbortLoiter -> ToLand : [abort_cmd == 0 && after(10, sec)]
    state Landcommand
      controlMode.land = 0;
    (default) -> Start
    Start -> (junction 5)
    FIXEDWINGFLIGHT -> WAYPOINT [order 2] : [(mode==2)]
        | {Status=uint8(0);}
    FIXEDWINGFLIGHT -> ORBIT [order 1] : [(mode==3)]
        | {Status= uint8(0);}
    (junction 262) -> FIXED_WING_ENTRY
    (junction 5) -> FIXED_WING_ORBIT [order 5] : [(mode==3)&&(FlightMode==flightState.FixedWing)]
        | {Status=uint8(0);}
    (junction 5) -> (junction 262) [order 3] : [(FlightMode==flightState.Transition)]
        | {controlMode.inTransition=0;}
    (junction 255) -> HOVER_ENTRY
    (junction 5) -> (junction 255) [order 4] : [(FlightMode==flightState.BackTransition)]
        | {controlMode.inTransition=0;}
    HOVER_ENTRY -> (junction 12)
    (junction 257) -> FIXED_WING_WAYPOINT
    Takeoff -> WP : [abs(Pose(3) - ToWP.position(3)) <= 1]{Status = 1;}
    RAMPUP -> Takeoff : [ramp_progress>=1.0]
    SPOOLUP -> RAMPUP : [spoolup_timer>=1.0]
    GuidanceLogic -> (junction 5) : [(hasChanged(mode))]
    (junction 5) -> SPOOLUP [order 7] : [(mode == 1)&&(FlightMode==flightState.Hover)]
        | {controlMode.inTransition=0;}
    (junction 5) -> (junction 257) [order 2] : [(mode==2)&&(FlightMode==flightState.FixedWing)]
        | {Status=uint8(0);}
    (junction 5) -> (junction 260) [order 1] : [(mode==6)&&(FlightMode==flightState.FixedWing)]
        | {courseHold=States.course;
        | altitudeHold=-States.Xe(3); }
    (junction 5) -> (junction 12) [order 6] : [FlightMode==flightState.Hover]
        | {controlMode.inTransition=0;}
    (junction 260) -> PreTransition
    (junction 12) -> WP [order 1] : [(mode==2)]
    (junction 12) -> (junction 17) [order 2]
    (junction 17) -> Orbit [order 1] : [(mode==3)]
    (junction 17) -> (junction 22) [order 2]
    PreTransition -> BackTransition : after(5,sec)
        | {FlightMode=flightState.BackTransition;
        | controlMode.inTransition=1;
        | controlMode.BackTransitionCondition = 0;
        | controlMode.attitude = 1;
        | controlMode.airspeedAltitude = 0;
        | controlMode.lateralGuidance = 0;}
    BackTransition -> BackCOMPLETE : [backConditioMet(States.airspeed, mc_weight)]
    (junction 22) -> ForwardTransition [order 1] : [(mode==6)]
        | {FlightMode=flightState.Transition;
        | controlMode.inTransition=1;
        | controlMode.attitude = 1;
        | controlMode.airspeedAltitude = 0;
        | controlMode.lateralGuidance = 0;
        | controlMode.TransitionCondition=uint8(0);
        | }
    (junction 22) -> Land [order 2] : [(mode == 4)]
    ForwardTransition -> FWCOMPLETE : [transitionConditionMet(mc_weight, States.airspeed, controlMode.inTransition)]
    Land -> Landcommand : [landDetected(States.Ve, States.pqr)]
  (default) -> GuidanceLogic
  data: sf_internal_action_state_placeholder_data local double size=1 =0; sf_internal_action_state_placeholder_data local double size=1 =0; sf_internal_action_state_placeholder_data local double size=1 =0; sf_internal_action_state_placeholder_data local double size=1 =0; sf_internal_action_state_placeholder_data local double size=1 =0; sf_internal_action_state_placeholder_data local double size=1 =0; sf_internal_action_state_placeholder_data local double size=1 =0; sf_internal_action_state_placeholder_data local double size=1 =0; sf_internal_action_state_placeholder_data local double size=1 =0; sf_internal_action_state_placeholder_data local double size=1 =0; Mc_weight function_input double; valid function_output; airspeed function_input; inTransition function_input; airspeed function_input; mc_weight function_input double; valid function_output; Ve function_input double; landed function_output; pqr function_input; mode input; ToWP input Bus: UAVPathManagerBus; Status output uint8; FromWP input Bus: UAVPathManagerBus; Pose input; GdncMode output Enum: GdncModeType; States input; aacSP output Bus: AAC; FixedWingSP output Bus: FixedWingCommandBus; controlMode output Bus: controlMode; FlightMode output; PresetMode input; courseHold local; altitudeHold local; Vt parameter double; InnerLoopCmds output Bus: innerLoopCmdsBus; zGround parameter; Ground input; mc_weight input; abort_cmd input boolean; ramp_progress local double; spoolup_timer local double
  function valid = transitionConditionMet(Mc_weight, airspeed, inTransition):
    | function valid = transitionConditionMet(Mc_weight, airspeed, inTransition)         
    |       %#codegen                                                                      
    |       % PX4-based forward transition completion check                                
    |       % mc_weight: unified MC weight (1=full MC, 0=full FW)                          
    |       % Conditions: time >= 30s AND airspeed >= 20 AND mc_weight <= 0                
    |       % Timeout fallback: 60s forced completion                                      
    | 
    |       DT_TRANS_SEC = 30.0;   % minimum transition time [s]
    |       DT_TRANS_MAX = 60.0;   % timeout: forced completion [s]
    |       V_TRANS      = 20.0;   % transition airspeed threshold [m/s]
    |       Ts           = 0.005;  % sample time [s]
    | 
    |       persistent dt_trans last_inTrans
    |       if isempty(dt_trans)
    |           dt_trans = 0.0;
    |           last_inTrans = uint8(0);
    |       end
    | 
    |       inT = uint8(inTransition > 0);
    | 
    |       % reset timer on rising edge (new transition entry)
    |       if (last_inTrans == 0) && (inT == 1)
    |           dt_trans = 0.0;
    |       end
    | 
    |       % accumulate elapsed time during transition
    |       if inT == 1
    |           dt_trans = dt_trans + Ts;
    |       else
    |           dt_trans = 0.0;
    |       end
    |       last_inTrans = inT;
    | 
    |       timeOK  = (dt_trans >= DT_TRANS_SEC);   % min time elapsed
    |       speedOK = (airspeed >= V_TRANS);         % airspeed reached
    |       modeOK  = (inT == 1);                   % currently in transition
    | 
    |       % normal: all conditions met (MC weight fully ramped down)
    |       normalComplete  = modeOK && timeOK && speedOK && (mc_weight <= 0.0);
    |       % timeout: forced completion after DT_TRANS_MAX
    |       timeoutComplete = modeOK && (dt_trans >= DT_TRANS_MAX);
    | 
    |       valid = normalComplete || timeoutComplete;
    |   end
  function valid = backConditioMet(airspeed, mc_weight):
    | function valid = backConditioMet(airspeed, mc_weight)
    |       %#codegen
    |       % mc_weight: unified MC weight (0=full FW, 1=full MC)
    |       % 3 OR conditions: weight ramp done | speed low | timeout
    | 
    |       V_BACK      = 4.0;    % speed threshold for MC mode [m/s]
    |       DT_BACK_MAX = 15.0;   % timeout: forced completion [s]
    |       Ts          = 0.005;  % sample time [s]
    | 
    |       persistent dt_back
    |       if isempty(dt_back)
    |           dt_back = 0.0;
    |       end
    | 
    |       % reset timer when still in FW (mc_weight near zero)
    |       if mc_weight <= 0.01
    |           dt_back = 0.0;
    |       end
    | 
    |       dt_back = dt_back + Ts;
    | 
    |       weightComplete = (mc_weight >= 0.99);   % MC weight fully ramped up
    |       speedComplete  = (airspeed < V_BACK);   % airspeed below MC threshold
    |       timeComplete   = (dt_back >= DT_BACK_MAX); % timeout fallback
    | 
    |       valid = weightComplete || speedComplete || timeComplete;
    |   end
  function landed = landDetected(Ve, pqr):
    | function landed = landDetected(Ve, pqr)
    |     %#codegen
    |     LNDMC_Z_VEL_MAX  = 0.5;    % 수직속도 임계 [m/s]
    |     LNDMC_XY_VEL_MAX = 2.0;     % 수평속도 임계 [m/s]
    |     LNDMC_ROT_MAX    = 30;      % 각속도 임계 [deg/s]
    |     LNDMC_TRIG_TIME  = 1.0;     % 판정 시간 [s] (기존 8초→1초)
    |     Ts               = 0.005;   % 샘플 시간 [s]
    | 
    |     persistent timer
    |     if isempty(timer), timer = 0.0; end
    | 
    |     vz_ok  = abs(Ve(3)) < LNDMC_Z_VEL_MAX;
    |     vxy_ok = sqrt(Ve(1)^2 + Ve(2)^2) < LNDMC_XY_VEL_MAX;
    |     rot_ok = sqrt(pqr(1)^2 + pqr(2)^2 + pqr(3)^2) * (180/pi) < LNDMC_ROT_MAX;
    | 
    |     maybe_landed = vz_ok && vxy_ok && rot_ok;
    | 
    |     if maybe_landed
    |         timer = timer + Ts;
    |     else
    |         timer = 0.0;
    |     end
    | 
    |     landed = (timer >= LNDMC_TRIG_TIME);
    | end

== matlab function untitled2/Guidance Mode Selector/GuidanceLogic.FIXED_WING_WAYPOINT.WAYPOINT/MATLAB Function ==
  data: toWP input; wps output; fromWP input; alt output
function [wps, alt]= fcn(toWP, fromWP)
    wps = zeros(2,3); %#ok<PREALL> 
    wps = [fromWP'; toWP'];
    alt = -toWP(3);
end

== matlab function untitled2/Guidance Mode Selector/GuidanceLogic.Land.Descend/MATLAB Function ==
  data: FromWP input Bus: UAVPathManagerBus size=1; wps output; ToWPPos input size=[3 1]; ToWPParam input size=[4 1]
function wps = getLandingWaypoint(FromWP, ToWPPos, ToWPParam)

persistent outWPS

if isempty(outWPS)
    outWPS = double(zeros(2,4));
end

outWPS(1,:) = [FromWP.position' FromWP.params(4)];
outWPS(2,:) = [reshape(ToWPPos,1,[]), ToWPParam(4)];

wps = outWPS;

== matlab function untitled2/Guidance Mode Selector/GuidanceLogic.Land.ToLand/MATLAB Function ==
  data: FromWP input Bus: UAVPathManagerBus size=1; wps output; ToWP input Bus: UAVPathManagerBus size=1
function wps = getLandingWaypoint(FromWP, ToWP)                                                                                 
    outWPS = double(zeros(2,4));                                                                                                  
    outWPS(1,:) = [FromWP.position' FromWP.params(1)];                                                                        
    outWPS(2,:) = [ToWP.position(1:2)' FromWP.position(3) ToWP.params(1)];
    wps = outWPS;
  end

== matlab function untitled2/Guidance Mode Selector/GuidanceLogic.WP/MATLAB Function ==
  data: FromWP input Bus: UAVPathManagerBus size=1; wps output; ToWP input Bus: UAVPathManagerBus size=1
function wps = getWaypointMission(FromWP, ToWP)

persistent outWPS

if isempty(outWPS)
    outWPS = double(zeros(2,4));
end

outWPS(1,:) = [FromWP.position' FromWP.params(1)];
outWPS(2,:) = [ToWP.position' ToWP.params(1)];

wps = outWPS;

== matlab function untitled2/Guidance Mode Selector/GuidanceLogic.Land.Descend/MATLAB Function3 ==
  data: Pose3 input; LAD output; ToWP3 input
function LAD = calcLookahead(Pose3, ToWP3)
    AGL = ToWP3 - Pose3;
    if AGL > 50
        LAD = 10;
    elseif AGL > 30
        LAD = 5+(AGL - 10)/6;    % 5m→5, 10m→15
    elseif AGL > 15
        LAD = 1 + (AGL - 1)/6;    % 1m→1, 5m→5
    else
        LAD = max(0.5, AGL * 1);    % 최소 0.5
    end
  end

== matlab function untitled2/Guidance Mode Selector/GuidanceLogic.Land.AbortLoiter/MATLAB Function ==
  data: FromWP input Bus: UAVPathManagerBus size=1; wps output; ToWPPos input size=[3 1]; ToWPParam input size=[4 1]
function wps = getLandingWaypoint(FromWP, ToWPPos, ToWPParam)

persistent outWPS

if isempty(outWPS)
    outWPS = double(zeros(2,4));
end

outWPS(1,:) = [FromWP.position' FromWP.params(4)];
outWPS(2,:) = [reshape(ToWPPos,1,[]), ToWPParam(4)];

wps = outWPS;

== matlab function untitled2/Guidance Mode Selector/GuidanceLogic.Land.Descend/MATLAB Function1 ==
  data: Pose3 input; LAD output; ToWP3 input
function LAD = calcLookahead(Pose3, ToWP3)
    AGL = ToWP3 - Pose3;
    if AGL > 50
        LAD = 2;
    elseif AGL > 30
        LAD = 2;    % 5m→5, 10m→15
    elseif AGL > 15
        LAD = 2;    % 1m→1, 5m→5
    else
        LAD = max(0.5, AGL * 1);    % 최소 0.5
    end
  end

== matlab function untitled2/Guidance Mode Selector/GuidanceLogic.Land.Descend/MATLAB Function2 ==
  data: LAP_in input; LAP_out output; Pose input; Ground input
function LAP_out = clampHorizontal(LAP_in, Pose, Ground)
    AGL = Ground - Pose(3);  % NED 좌표계

    if AGL < 0.5
        LAP_out = LAP_in;
        LAP_out(1) = Pose(1);  % X → 현재 위치
        LAP_out(2) = Pose(2);   % Y → 현재 위치
        
    else
        LAP_out = LAP_in;
    end
  end
